simulink model "hdl_learn_fir"  (R2025b)
settings: Solver=FixedStepDiscrete  StartTime=0.0  StopTime=0.05  FixedStep=0.0001  RelTol=1e-3
libraries: simulink x1
settings Model: DataTypeOverride=Off  Creator=kimsteph  LastModifiedBy=kimsteph
settings OptimizationCC: BlockReduction=off  ConditionallyExecuteInputs=off  DefaultParameterBehavior=Inlined  InheritOutputTypeSmallerThanSingle=on
settings DebuggingCC: ArtificialAlgebraicLoopMsg=error  SingleTaskRateTransMsg=error
settings HardwareCC: ProdBitPerPointer=32.0  ProdBitPerSizeT=32.0  ProdBitPerPtrDiffT=32.0  ProdLargestAtomicFloat=None  ProdIntDivRoundTo=Undefined  ProdEndianess=Unspecified  ProdWordSize=32.0  ProdHWDeviceType=ASIC/FPGA->ASIC/FPGA  TargetBitPerPointer=64.0  TargetBitPerSizeT=64.0  TargetBitPerPtrDiffT=64.0  TargetLongLongMode=on  TargetIntDivRoundTo=Zero  TargetEndianess=LittleEndian  TargetWordSize=64.0  TargetHWDeviceType=Custom Processor->MATLAB Host Computer  ProdEqTarget=off

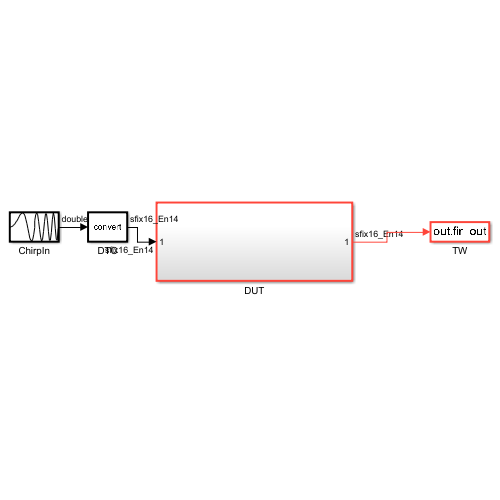
[thumbnail: Simulink's stored preview of the top-level diagram]
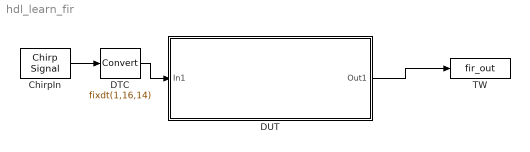
== system hdl_learn_fir ==
  ChirpIn : simulink/Sources/Chirp Signal  f1=100  T=0.05  f2=2000
  DTC : DataTypeConversion  OutDataTypeStr=fixdt(1,16,14)  RndMeth=Nearest  SaturateOnIntegerOverflow=off
  DUT : Subsystem
  TW : ToWorkspace  VariableName=fir_out  SaveFormat=Timeseries  SampleTime=-1
  wires:
  ChirpIn/1 -> DTC/1
  DTC/1 -> DUT/1(In1)
  DUT/1(Out1) -> TW/1

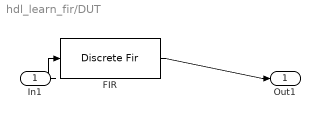
== system hdl_learn_fir/DUT ==
  In1 : Inport  OutDataTypeStr=fixdt(1,16,14)
  FIR : DiscreteFir  Coefficients=[0.02802 0.09763 0.166 0.2083 0.2083 0.166 0.09763 0.02802]  SampleTime=0.0001  CoefDataTypeStr=fixdt(1,16,14)  ProductDataTypeStr=fixdt(1,32,28)  AccumDataTypeStr=fixdt(1,32,28)  OutDataTypeStr=fixdt(1,16,14)
  Out1 : Outport
  wires:
  In1/1 -> FIR/1
  FIR/1 -> Out1/1
